simulink library "FadeControl"  (R2022b)
settings: Solver=VariableStepAuto  StartTime=0.0  StopTime=10.0  RelTol=1e-3
libraries: FadeControlBtc x1
settings Model: Creator=db1045444  LastModifiedBy=kl13806
settings SolverCC: AlgebraicLoopSolver=TrustRegion
settings DebuggingCC: UnconnectedInputMsg=warning  UnconnectedOutputMsg=warning  UnconnectedLineMsg=warning  SFMachineParentedDataDiag=warning
settings ModelReferenceCC: EnableRefExpFcnMdlSchedulingChecks=on
settings RTWCC: DLArmComputeVersion=19.05

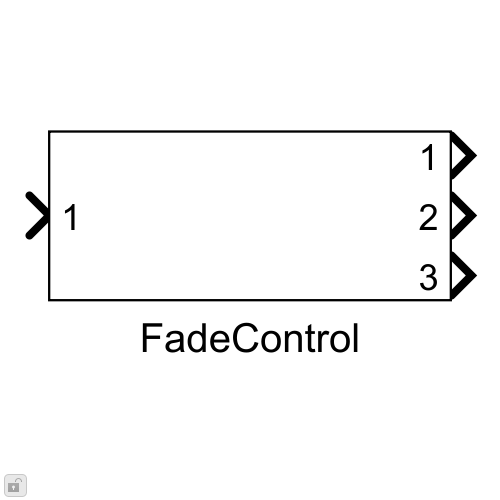
[thumbnail: Simulink's stored preview of the top-level diagram]
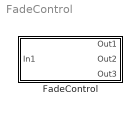
== system FadeControl ==
  FadeControl : Subsystem  mask(Bose FadeControl){MaskIndexOffset=128, MaskBoostDisable=off, MaskSilentExtreme=on, BankNumber=0}
      mask prompts: MaskIndexOffset "Index Offset"; MaskBoostDisable "Disable Boost"; MaskSilentExtreme "Enable Silent Extreme"; BankNumber "Target Memory Bank Number"
      mask help: This component is to be used in conjunction with 1 or more instances of the FadeRamper block. It provides the control layer for Fade processing via an RTC and tune variables.
      mask init:
      | blkh = gcbh;
      | % Copy discrete mask parameters into a classdef object
      | InnerLinkConfig = FadeControlConfig;
      | InnerLinkConfig.DefaultIndexOffset = MaskIndexOffset;
      | InnerLinkConfig.DefaultBoostDisable = MaskBoostDisable;
      | InnerLinkConfig.DefaultSilentExtreme = MaskSilentExtreme;
      | InnerLinkConfig.BankNumber = BankNumber;
      mask Help: If this control block is being used in a "multi-instance" manner, i.e. it is contorlling two or more FadeRamper blocks, there is an additional step that must be done. The developer must add a function-triggered subsytem containing an AND logic gate, which will combine the notification completion signals of the multiple ramper instances. The output of this subsytem must then feed the NTF_done input of the FadeControl block.

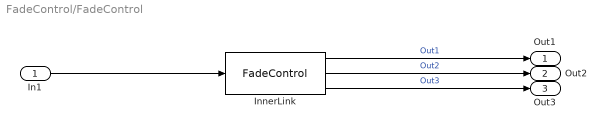
== system FadeControl/FadeControl ==
  In1 : Inport
  InnerLink : FadeControlBtc/FadeControl  Config=InnerLinkConfig  FeatureName=FadeControl
      settings: SourceProductName=Bose Blocklib
  Out1 : Outport
  Out2 : Outport  Port=2
  Out3 : Outport  Port=3
  wires:
  InnerLink/1 -> Out1/1  "Out1"
  InnerLink/2 -> Out2/1  "Out2"
  InnerLink/3 -> Out3/1  "Out3"
  In1/1 -> InnerLink/1
